simulink model "sync_flier_modelling_non_d"  (R2024a)
settings: Solver=FixedStepAuto  StartTime=0.0  StopTime=500  FixedStep=dt  RelTol=1e-3
values from neighbouring files (symbols this model uses):
  kd = MT*0.5    [Generate_Lambda_stiffness_sync.m]    (also in Generate_bumblebee_data.m = 0.29; Generate_data_Emergent_time_amplitude.m = 0.5; Generate_data_async.m = 0.5; Generate_data_at_different_lambda_stiff_for_Fig_5.m)
  kt = 1 - ku - kd    (= 0)    [Generate_Lambda_stiffness_sync.m]    (also in Generate_bumblebee_data.m = 0.42; Generate_data_Emergent_time_amplitude.m; Generate_data_async.m; Generate_data_at_different_lambda_stiff_for_Fig_5.m)
  ku = MT*0.5    [Generate_Lambda_stiffness_sync.m]    (also in Generate_bumblebee_data.m = 0.29; Generate_data_Emergent_time_amplitude.m = 0.5; Generate_data_async.m = 0.5; Generate_data_at_different_lambda_stiff_for_Fig_5.m)
  P1 = P1allfinal(Indices(p1i))    [Generate_Lambda_stiffness_sync.m]    (also in Generate_bumblebee_data.m = 0.75; Generate_consolidated_and_thorax_data_sync_no_spring.m = P1allfinal(1,p1i); Generate_data_Emergent_time_amplitude.m = P1allnew(1,p1i); Generate_data_async.m = P1allnew(1,p1i))
  P2 = P2new(Indices(p1i))    [Generate_Lambda_stiffness_sync.m]    (also in Generate_bumblebee_data.m = P2_bumblebee*Achange_all(1,ai); Generate_consolidated_and_thorax_data_sync_no_spring.m = P2new(1,p1i); Generate_data_async.m = P2new(1,p1i); Generate_data_at_different_lambda_stiff_for_Fig_5.m)
  P3 = P3all(1,p3i)    [Generate_Lambda_stiffness_sync.m]    (also in Generate_consolidated_and_thorax_data_sync_no_spring.m = P3all(p3i); Generate_data_at_different_lambda_stiff_for_Fig_5.m; Generate_data_at_different_lambda_stiff_for_async.m = 1; Generate_data_at_different_lambda_stiff_for_sync.m)
  xt = 0    [Generate_Lambda_stiffness_sync.m]    (also in Generate_bumblebee_data.m; Generate_data_Emergent_time_amplitude.m; Generate_data_async.m; Generate_data_at_different_lambda_stiff_for_Fig_5.m)
libraries: simulink x4
settings Model: Creator=suyash  LastModifiedBy=suyash
settings SolverCC: ZeroCrossAlgorithm=Adaptive
settings DebuggingCC: UnconnectedInputMsg=warning  UnconnectedOutputMsg=warning  UnconnectedLineMsg=warning
settings ModelReferenceCC: EnableRefExpFcnMdlSchedulingChecks=on
settings RTWCC: GPUComputeCapability=3.5  DLArmComputeVersion=19.05

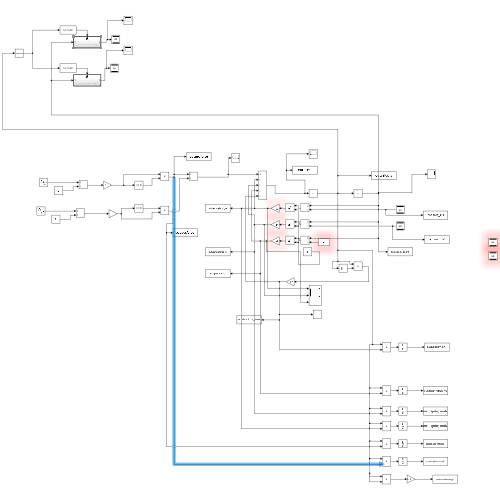
[thumbnail: Simulink's stored preview of the top-level diagram]
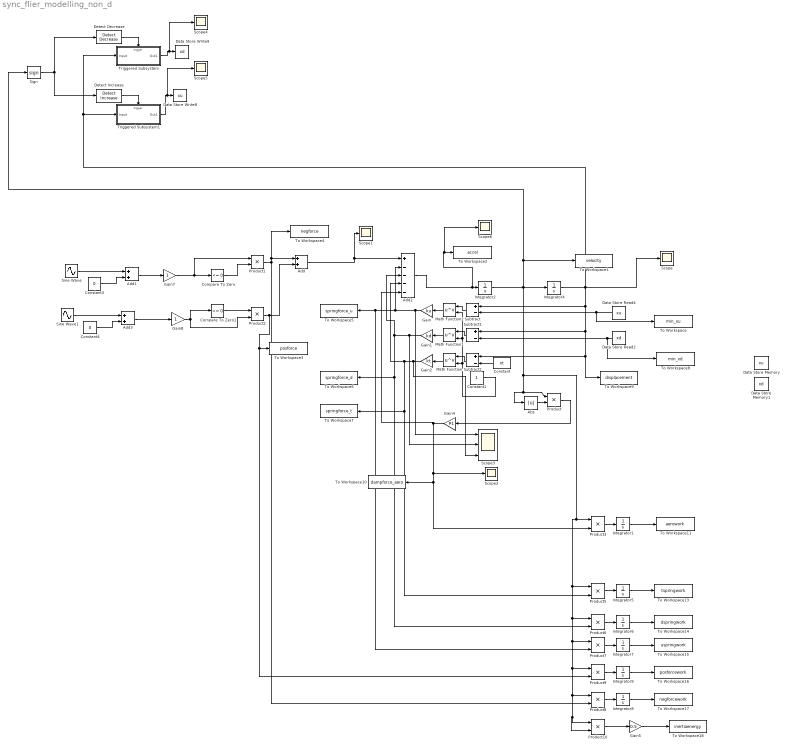
== system sync_flier_modelling_non_d ==
  Abs : Abs  SaturateOnIntegerOverflow=off
  Add : Sum
  Add1 : Sum
  Add2 : Sum  Inputs=+----
  Add3 : Sum
  Compare To Zero : simulink/Logic and Bit Operations/Compare To Zero  relop=<=  OutDataTypeStr=boolean
  Compare To Zero1 : simulink/Logic and Bit Operations/Compare To Zero  relop=>=  OutDataTypeStr=boolean
  Constant : Constant  Value=xt
  Constant1 : Constant
  Constant3 : Constant  Value=0
  Constant4 : Constant  Value=0
  Data Store Memory : DataStoreMemory  DataStoreName=xu  ReadBeforeWriteMsg=warning  WriteAfterWriteMsg=warning  WriteAfterReadMsg=warning  InitialValue=xu_min  ShowAdditionalParam=off
  Data Store Memory1 : DataStoreMemory  DataStoreName=xd  ReadBeforeWriteMsg=warning  WriteAfterWriteMsg=warning  WriteAfterReadMsg=warning  InitialValue=xd_max  ShowAdditionalParam=off
  Data Store Read2 : DataStoreRead  DataStoreName=xd  IndexOptions=Index vector (dialog)  Indices=1  OutputSizes=1
  Data Store Read4 : DataStoreRead  DataStoreName=xu  IndexOptions=Index vector (dialog)  Indices=1  OutputSizes=1
  Data Store Write8 : DataStoreWrite  DataStoreName=xu  IndexOptions=Index vector (dialog)  Indices=1  OutputSizes=1
  Data Store Write9 : DataStoreWrite  DataStoreName=xd  IndexOptions=Index vector (dialog)  Indices=1  OutputSizes=1
  Detect Decrease : simulink/Logic and Bit Operations/Detect Decrease  vinit=0.0  OutDataTypeStr=boolean
  Detect Increase : simulink/Logic and Bit Operations/Detect Increase  vinit=0.0  OutDataTypeStr=boolean
  Gain : Gain  Gain=ku
  Gain1 : Gain  Gain=kd
  Gain2 : Gain  Gain=kt
  Gain4 : Gain  Gain=P1
  Gain5 : Gain  Gain=0.5
  Gain7 : Gain
  Gain8 : Gain
  Integrator{1,4..9} (7 alike) : Integrator
  Integrator2 : Integrator  InitialCondition=1
  Math Function : Math  Operator=pow
  Math Function1 : Math  Operator=pow
  Math Function2 : Math  Operator=pow
  Product{,1..3,5..10} (10 alike) : Product
  Scope{,1..2,4..6} (6 alike) : Scope
  Scope3 : Scope  NumInputPorts=3
  Sign : Signum
  Sine Wave : Sin  Amplitude=P2  Frequency=P3  SampleTime=0
  Sine Wave1 : Sin  Amplitude=P2  Frequency=P3  SampleTime=0
  Subtract : Sum  Inputs=+-
  Subtract1 : Sum  Inputs=+-
  Subtract2 : Sum  Inputs=+-
  To Workspace : ToWorkspace  VariableName=min_xu  SaveFormat=Timeseries  SampleTime=-1
  To Workspace1 : ToWorkspace  VariableName=velocity  SaveFormat=Timeseries  SampleTime=-1
  To Workspace10 : ToWorkspace  VariableName=dampforce_aero  SaveFormat=Timeseries  SampleTime=-1
  To Workspace11 : ToWorkspace  VariableName=aerowork  SaveFormat=Timeseries  SampleTime=-1
  To Workspace13 : ToWorkspace  VariableName=tspringwork  SaveFormat=Timeseries  SampleTime=-1
  To Workspace14 : ToWorkspace  VariableName=dspringwork  SaveFormat=Timeseries  SampleTime=-1
  To Workspace15 : ToWorkspace  VariableName=uspringwork  SaveFormat=Timeseries  SampleTime=-1
  To Workspace16 : ToWorkspace  VariableName=posforcework  SaveFormat=Timeseries  SampleTime=-1
  To Workspace17 : ToWorkspace  VariableName=negforcework  SaveFormat=Timeseries  SampleTime=-1
  To Workspace18 : ToWorkspace  VariableName=inertiaenergy  SaveFormat=Timeseries  SampleTime=-1
  To Workspace2 : ToWorkspace  VariableName=accel  SaveFormat=Timeseries  SampleTime=-1
  To Workspace3 : ToWorkspace  VariableName=posforce  SaveFormat=Timeseries  SampleTime=-1
  To Workspace4 : ToWorkspace  VariableName=negforce  SaveFormat=Timeseries  SampleTime=-1
  To Workspace5 : ToWorkspace  VariableName=springforce_u  SaveFormat=Timeseries  SampleTime=-1
  To Workspace6 : ToWorkspace  VariableName=springforce_d  SaveFormat=Timeseries  SampleTime=-1
  To Workspace7 : ToWorkspace  VariableName=springforce_t  SaveFormat=Timeseries  SampleTime=-1
  To Workspace8 : ToWorkspace  VariableName=min_xd  SaveFormat=Timeseries  SampleTime=-1
  To Workspace9 : ToWorkspace  VariableName=displacement  SaveFormat=Timeseries  SampleTime=-1
  Triggered Subsystem : Subsystem  TreatAsAtomicUnit=on
  Triggered Subsystem1 : Subsystem  TreatAsAtomicUnit=on
  wires:
  Subtract2/1 -> Math Function/1
  Constant/1 -> Subtract2/2
  Product/1 -> Gain4/1
  Abs/1 -> Product/2
  Data Store Read2/1 -> To Workspace8/1, Subtract1/2
  Data Store Read4/1 -> To Workspace/1, Subtract/2
  Integrator7/1 -> To Workspace15/1
  Integrator9/1 -> To Workspace16/1
  Integrator6/1 -> To Workspace14/1
  Gain4/1 -> Add2/5, Scope2/1, Product3/2, To Workspace10/1
  Integrator8/1 -> To Workspace17/1
  Product8/1 -> Integrator8/1
  Product9/1 -> Integrator9/1
  Product7/1 -> Integrator7/1
  Gain2/1 -> Scope3/3, To Workspace7/1, Product5/2, Add2/4
  Gain1/1 -> Scope3/2, Product6/2, To Workspace6/1, Add2/3
  Integrator1/1 -> To Workspace11/1
  Product10/1 -> Gain5/1
  Product3/1 -> Integrator1/1
  Integrator5/1 -> To Workspace13/1
  Product6/1 -> Integrator6/1
  Gain5/1 -> To Workspace18/1
  Gain/1 -> Product7/2, To Workspace5/1, Add2/2, Scope3/1
  Product5/1 -> Integrator5/1
  Add2/1 -> Scope6/1, To Workspace2/1, Integrator2/1
  Gain7/1 -> Compare To Zero/1, Product1/1
  Gain8/1 -> Product2/2, Compare To Zero1/1
  Constant3/1 -> Add1/2
  Sine Wave/1 -> Add1/1
  Add1/1 -> Gain7/1
  Product2/1 -> Product9/2, To Workspace3/1, Add/2
  Product1/1 -> To Workspace4/1, Add/1, Product8/2
  Add3/1 -> Gain8/1
  Sine Wave1/1 -> Add3/1
  Constant4/1 -> Add3/2
  Compare To Zero/1 -> Product1/2
  Compare To Zero1/1 -> Product2/1
  Sign/1 -> Detect Increase/1, Detect Decrease/1
  Detect Decrease/1 -> Triggered Subsystem/Trigger
  Detect Increase/1 -> Triggered Subsystem1/Trigger
  Triggered Subsystem1/1(Out1) -> Scope5/1, Data Store Write8/1
  Integrator2/1 -> Sign/1, To Workspace1/1, Integrator4/1, Product10/2, Product10/1, Product8/1, Product9/1, Product7/1, Product6/1, Product5/1, Product3/1, Abs/1, Product/1
  Integrator4/1 -> Scope/1, Triggered Subsystem1/1(Input), Triggered Subsystem/1(Input), To Workspace9/1, Subtract2/1, Subtract1/1, Subtract/1
  Triggered Subsystem/1(Out1) -> Scope4/1, Data Store Write9/1
  Add/1 -> Scope1/1, Add2/1
  Constant1/1 -> Math Function1/2, Math Function2/2, Math Function/2
  Math Function/1 -> Gain2/1
  Math Function2/1 -> Gain/1
  Math Function1/1 -> Gain1/1
  Subtract1/1 -> Math Function1/1
  Subtract/1 -> Math Function2/1

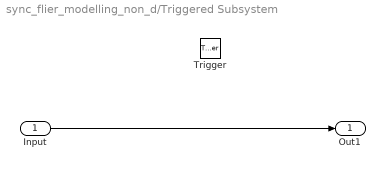
== system sync_flier_modelling_non_d/Triggered Subsystem ==
  Input : Inport
  Trigger : TriggerPort  VariantControl=(inherit)
  Out1 : Outport
  wires:
  Input/1 -> Out1/1

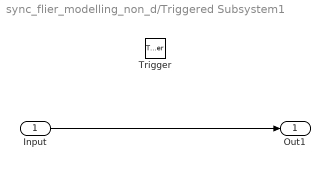
== system sync_flier_modelling_non_d/Triggered Subsystem1 ==
  Input : Inport
  Trigger : TriggerPort  VariantControl=(inherit)
  Out1 : Outport
  wires:
  Input/1 -> Out1/1
